simulink model "L2_Q1_Sim"  (R2015a)
settings: Solver=ode3  StartTime=0.0  StopTime=tf  FixedStep=t_step  RelTol=1e-3
values from neighbouring files (symbols this model uses):
  K0 = (4/ts)^2 + (4*pi/(ts*log(Mp)))^2    [L2_Q1.m]    (also in L2_Q2.m; L2_Q3.m)
  K1 = 8 / ts    (= 8)    [L2_Q1.m]    (also in L2_Q2.m; L2_Q3.m)
  r = 5    [L2_Q1.m]
settings Model: Creator=Marcelo  LastModifiedBy=Marcelo

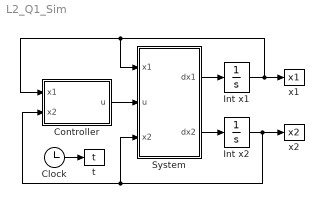
== system L2_Q1_Sim ==
  Clock : Clock
  Controller : MATLAB Function  TreatAsAtomicUnit=on
  Int x1 : Integrator
  Int x2 : Integrator
  System : MATLAB Function  TreatAsAtomicUnit=on
  t : ToWorkspace  VariableName=t  SampleTime=-1
  x1 : ToWorkspace  VariableName=x1  SampleTime=-1
  x2 : ToWorkspace  VariableName=x2  SampleTime=-1
  wires:
  Clock/1 -> t/1
  Int x2/1 -> Controller/2(x2), System/3(x2), x2/1
  Int x1/1 -> System/1(x1), Controller/1(x1), x1/1
  System/2(dx2) -> Int x2/1
  System/1(dx1) -> Int x1/1
  Controller/1(u) -> System/2(u)

== matlab function L2_Q1_Sim/System ==
  data: x1 input; u input; dx1 output; dx2 output; x2 input
function [dx1, dx2] = fcn(x1, u, x2)
dx1 = x1^2 + x2;
dx2 = u;

== matlab function L2_Q1_Sim/Controller ==
  data: u output; x1 input; x2 input; K1 parameter; K0 parameter; r parameter
function u = fcn(x1, x2, K1, K0, r)
v = - K1 * (x1^2 + x2) - K0 * (x1 - r);
u = v - 2*x1^3 - 2*x1*x2;
